simulink model "FOC_Part2"  (R2021b)
settings: Solver=ode45  StartTime=0.0  StopTime=0.2  MaxStep=1e-6  RelTol=1e-3
undefined symbols (not defined in the file): CurKi, CurKp, CurMax, CurTs, F, Id_Target, J, Kt, Ld, Lq, Ls, Mode, Np, Rs, SpdKi, SpdKp, SpdTs, TargetSpd, Tf, Theta_Init, TickAdd, Tn, Udc, VolMax
libraries: spsPermanentMagnetSynchronousMachineLib x1, spsCurrentMeasurementLib x1, spsDCVoltageSourceLib x1, eeGeneralControl x1, spsOnDelayLib x1, simulink x1, spsUniversalBridgeLib x1, spsVoltageMeasurementLib x1, spspowerguiLib x1
settings Model: SimulationMode=accelerator  Creator=LFL  LastModifiedBy=62555
settings SolverCC: AlgebraicLoopSolver=TrustRegion
settings DataIOCC: ReturnWorkspaceOutputs=off
settings DebuggingCC: SFMachineParentedDataDiag=warning  ArithmeticOperatorsInVariantConditions=warning
settings SFSimCC: SimUseLocalCustomCode=off  CustomCodeUndefinedFunction=UseInterfaceOnly
settings RTWCC: RTWUseLocalCustomCode=off

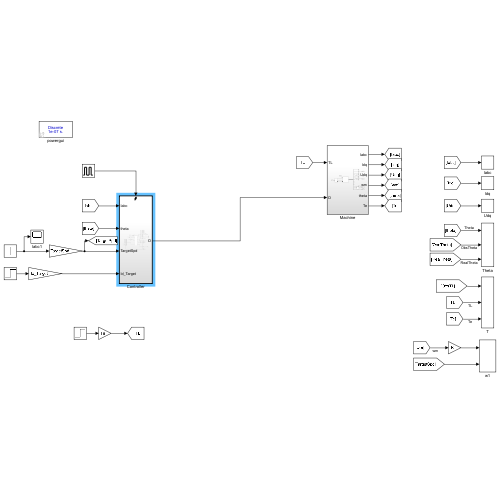
[thumbnail: Simulink's stored preview of the top-level diagram]
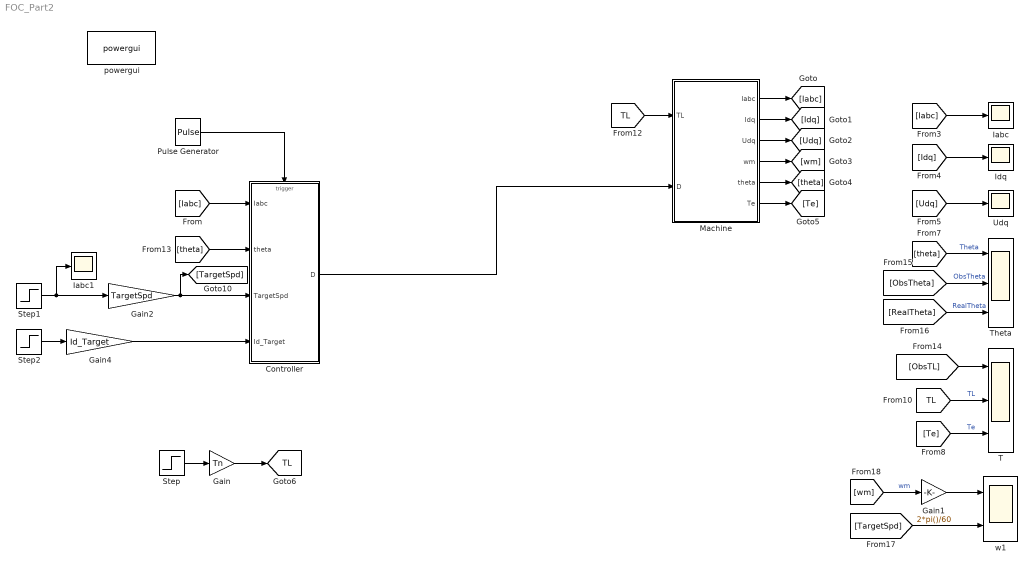
== system FOC_Part2 ==
  Controller : Subsystem  TreatAsAtomicUnit=on
  Gain : Gain  Gain=Tn
  Gain1 : Gain  Gain=2*pi()/60
  Gain2 : Gain  Gain=TargetSpd
  Gain4 : Gain  Gain=Id_Target
  Iabc : Scope
  Iabc1 : Scope
  Idq : Scope
  Machine : Subsystem
  Pulse Generator : DiscretePulseGenerator  PulseType=Time based  Period=CurTs  PulseWidth=50
  Step : Step  Time=0  SampleTime=0
  Step1 : Step  Time=0.1  SampleTime=0
  Step2 : Step  Time=0.1  SampleTime=0
  T : Scope  NumInputPorts=3
  Theta : Scope  NumInputPorts=3
  Udq : Scope
  powergui : spspowerguiLib/powergui  Priority=1  SimulationMode=Discrete  SampleTime=1/500/20000  frequency=60  Iterations=50  frequencyindice=0  Pbase=100e6  ErrMax=1e-4  UnitsV=kV  UnitsW=MW  buscounter=0  FunctionMessages=off  echomessages=off  EnableUseOfTLC=off  CurrentSourceSwitches=off  DisableSnubberDevices=off  DisableRonSwitches=off  DisableVfSwitches=off  DisplayEquations=off  AutomaticDiscreteSolvers=off  SolverType=Tustin/Backward Euler (TBE)  Interpol=off  ExternalGateDelay=off  methode=off  Ts=100  x0status=blocks  SPID=on  SwTol=0  HookPort=off  NonlinearTolerance=1e-4  nMaxIteration=100  ContinueOnMaxIteration=off  RestoreLinks=warning  ResistiveCurrentMeasurement=off  Frange=[0:2:500]  Ylog=off  Xlog=on  ShowGrid=off  save=off  variable=ZData  structure=0  ZoomFFT=off  StartTime=0.0  cycles=1  DisplayStyle=1  fundamental=60  FreqAxis=off  MaxFrequency=1000  frequencyindicesteady=1  RmsSteady=1  display=off
  w1 : Scope  NumInputPorts=2
  tag scope: TL=global
  wires:
  Pulse Generator/1 -> Controller/Trigger
  Machine/1(Iabc) -> [Iabc]
  Machine/2(Idq) -> [Idq]
  Machine/3(Udq) -> [Udq]
  Machine/4(wm) -> [wm]
  Machine/5(theta) -> [theta]
  Machine/6(Te) -> [Te]
  [Iabc] -> Controller/1(Iabc)
  [Iabc] -> Iabc/1
  [Udq] -> Udq/1
  [TL] -> T/2  "TL"
  [Te] -> T/3  "Te"
  [theta] -> Theta/1  "Theta"
  [Idq] -> Idq/1
  [TL] -> Machine/1(TL)
  [theta] -> Controller/2(theta)
  Step/1 -> Gain/1
  Gain/1 -> [TL]
  Controller/1(D) -> Machine/2(D)
  Gain2/1 -> Controller/3(TargetSpd), [TargetSpd]
  [ObsTL] -> T/1
  [ObsTheta] -> Theta/2  "ObsTheta"
  [RealTheta] -> Theta/3  "RealTheta"
  Step1/1 -> Gain2/1, Iabc1/1
  [TargetSpd] -> w1/2
  [wm] -> Gain1/1  "wm"
  Gain1/1 -> w1/1
  Step2/1 -> Gain4/1
  Gain4/1 -> Controller/4(Id_Target)

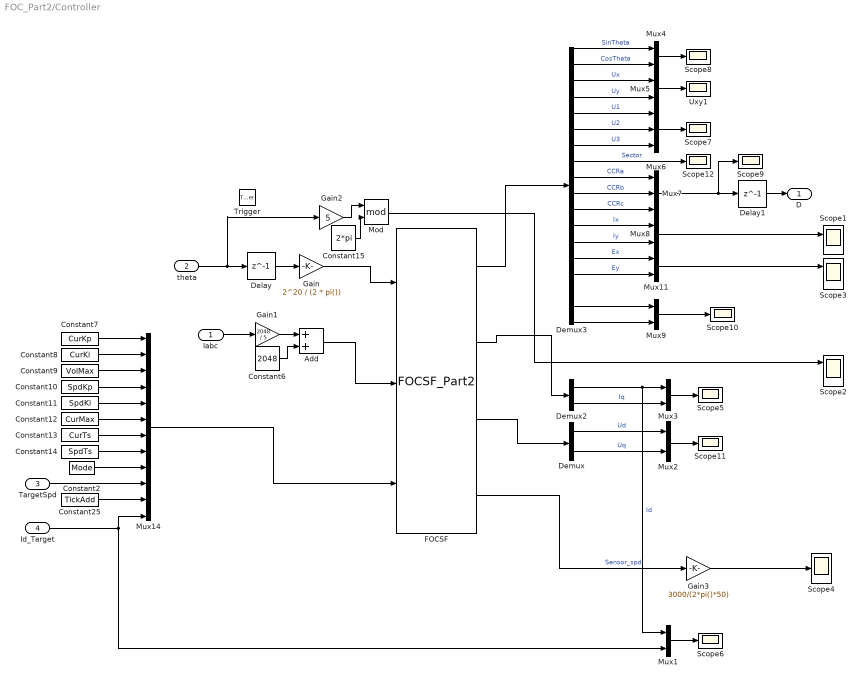
== system FOC_Part2/Controller ==
  Iabc : Inport
  theta : Inport  Port=2
  TargetSpd : Inport  Port=3
  Id_Target : Inport  Port=4
  Trigger : TriggerPort  VariantControl=Variant
  Add : Sum
  Constant10 : Constant  Value=SpdKp
  Constant11 : Constant  Value=SpdKi
  Constant12 : Constant  Value=CurMax
  Constant13 : Constant  Value=CurTs
  Constant14 : Constant  Value=SpdTs
  Constant15 : Constant  Value=2*pi
  Constant2 : Constant  Value=Mode
  Constant25 : Constant  Value=TickAdd
  Constant6 : Constant  Value=2048
  Constant7 : Constant  Value=CurKp
  Constant8 : Constant  Value=CurKi
  Constant9 : Constant  Value=VolMax
  Delay : Delay  DelayLength=1
  Delay1 : Delay  DelayLength=1
  Demux : Demux  Outputs=2
  Demux2 : Demux  Outputs=2
  Demux3 : Demux  Outputs=18
  FOCSF : S-Function  FunctionName=FOCSF_Part2  Parameters=Np Udc Ls Rs Kt J Ld Lq  SFunctionDeploymentMode=off  EnableBusSupport=off  mask{Np=Np, Udc=Udc, Ls=Ls, Rs=Rs, Kt=Kt, J=J, Ld=Ld, Lq=Lq}
      mask Display:
      | port_label('input',  1,  'Theta')
      | port_label('input',  2,  'Iabc')
      | port_label('input',  3,  'CtrlParam')
      | port_label('output', 1,  'FOC')
      | port_label('output', 2,  'Idq')
      | port_label('output', 3,  'Udq')
      | port_label('output', 4,  'Spd')
  Gain : Gain  Gain=2^20 / (2 * pi())
  Gain1 : Gain  Gain=2048 / 5
  Gain2 : Gain  Gain=5
  Gain3 : Gain  Gain=3000/(2*pi()*50)
  Mod : Math  Operator=mod  SaturateOnIntegerOverflow=on
  Mux{1..5,8..9,11} (8 alike) : Mux  Inputs=2
  Mux14 : Mux  Inputs=12
  Mux6 : Mux  Inputs=3
  Mux7 : Mux  Inputs=3
  Scope1 : Scope  NumInputPorts=2
  Scope{4..12} (9 alike) : Scope
  Scope2 : Scope  NumInputPorts=2
  Scope3 : Scope  NumInputPorts=2
  Uxy1 : Scope
  D : Outport  VectorParamsAs1DForOutWhenUnconnected=off
  wires:
  Iabc/1 -> Gain1/1
  Gain/1 -> FOCSF/1
  Gain1/1 -> Add/1
  Constant6/1 -> Add/2
  Add/1 -> FOCSF/2
  theta/1 -> Gain2/1, Delay/1
  Delay/1 -> Gain/1
  FOCSF/2 -> Demux2/1
  FOCSF/3 -> Demux/1
  Demux/1 -> Mux2/1  "Ud"
  Demux/2 -> Mux2/2  "Uq"
  Mux2/1 -> Scope11/1
  Delay1/1 -> D/1
  Demux2/1 -> Mux1/1, Mux3/1  "Id"
  Demux2/2 -> Mux3/2  "Iq"
  Mux3/1 -> Scope5/1
  FOCSF/1 -> Demux3/1
  Demux3/1 -> Mux4/1  "SinTheta"
  Demux3/2 -> Mux4/2  "CosTheta"
  Mux4/1 -> Scope8/1
  Demux3/3 -> Mux5/1  "Ux"
  Demux3/4 -> Mux5/2  "Uy"
  Mux6/1 -> Scope7/1
  Demux3/5 -> Mux6/1  "U1"
  Demux3/6 -> Mux6/2  "U2"
  Demux3/7 -> Mux6/3  "U3"
  Demux3/8 -> Scope12/1  "Sector"
  Demux3/9 -> Mux7/1  "CCRa"
  Demux3/10 -> Mux7/2  "CCRb"
  Demux3/11 -> Mux7/3  "CCRc"
  Mux7/1 -> Scope9/1, Delay1/1
  Demux3/13 -> Mux8/2  "Iy"
  Demux3/12 -> Mux8/1  "Ix"
  Demux3/15 -> Mux11/2  "Ey"
  Demux3/14 -> Mux11/1  "Ex"
  Mux14/1 -> FOCSF/3
  Constant7/1 -> Mux14/1
  Constant8/1 -> Mux14/2
  Constant9/1 -> Mux14/3
  Constant11/1 -> Mux14/5
  Constant10/1 -> Mux14/4
  Constant12/1 -> Mux14/6
  Constant13/1 -> Mux14/7
  Constant14/1 -> Mux14/8
  Constant2/1 -> Mux14/9
  TargetSpd/1 -> Mux14/10
  Constant25/1 -> Mux14/11
  Mux5/1 -> Uxy1/1
  Mux11/1 -> Scope3/1
  Mux8/1 -> Scope1/1
  Gain2/1 -> Mod/1
  Mod/1 -> Scope2/1
  Constant15/1 -> Mod/2
  FOCSF/4 -> Gain3/1  "Sensor_spd"
  Id_Target/1 -> Mux1/2, Mux14/12
  Mux1/1 -> Scope6/1
  Gain3/1 -> Scope4/1
  Demux3/17 -> Mux9/1
  Demux3/18 -> Mux9/2
  Mux9/1 -> Scope10/1

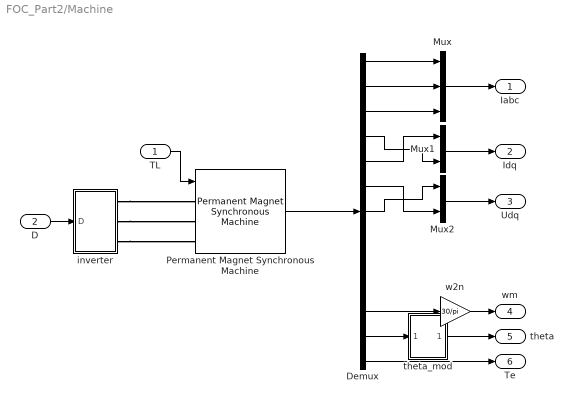
== system FOC_Part2/Machine ==
  TL : Inport
  D : Inport  Port=2
  Demux : Demux  Outputs=13
  Mux : Mux  Inputs=3
  Mux1 : Mux  Inputs=2
  Mux2 : Mux  Inputs=2
  Permanent Magnet Synchronous Machine : spsPermanentMagnetSynchronousMachineLib/Permanent Magnet Synchronous Machine  NbPhases=3  FluxDistribution=Sinusoidal  RotorType=Salient-pole  MechanicalLoad=Torque Tm  PresetModel=No  ShowDetailedParameters=on  MeasurementBus=off  Resistance=Rs  Inductance=8.5e-3  dqInductances=[Ld, Lq]  La=0.000395  MachineConstant=Torque Constant (N.m / A_peak)  Flux=0.014667  VoltageCst=13.3012  TorqueCst=Kt  Flat=120  Mechanical=[J F Np Tf]  PolePairs=4  InitialConditions=[0,Theta_Init, 0,0]  InitialConditions5ph=[0 0 0 0 0 0]  RefAngle=Aligned with phase A axis (original Park)  IterativeDiscreteModel=Trapezoidal non iterative  TsBlock=-1  TsPowergui=0
  inverter : Subsystem
  theta_mod : Subsystem
  w2n : Gain  Gain=30/pi
  Iabc : Outport  VectorParamsAs1DForOutWhenUnconnected=off
  Idq : Outport  Port=2  VectorParamsAs1DForOutWhenUnconnected=off
  Udq : Outport  Port=3  VectorParamsAs1DForOutWhenUnconnected=off
  wm : Outport  Port=4  VectorParamsAs1DForOutWhenUnconnected=off
  theta : Outport  Port=5  VectorParamsAs1DForOutWhenUnconnected=off
  Te : Outport  Port=6  VectorParamsAs1DForOutWhenUnconnected=off
  wires:
  Permanent Magnet Synchronous Machine/1 -> Demux/1
  Demux/1 -> Mux/1
  Demux/2 -> Mux/2
  Demux/3 -> Mux/3
  Mux/1 -> Iabc/1
  Mux1/1 -> Idq/1
  Mux2/1 -> Udq/1
  Demux/11 -> w2n/1
  Demux/12 -> theta_mod/1(In1)
  Demux/13 -> Te/1
  TL/1 -> Permanent Magnet Synchronous Machine/1
  Demux/5 -> Mux1/1
  Demux/4 -> Mux1/2
  Demux/6 -> Mux2/2
  Demux/7 -> Mux2/1
  theta_mod/1(Out1) -> theta/1
  w2n/1 -> wm/1
  D/1 -> inverter/1(D)
  connections:
  inverter/RConn1 -- Permanent Magnet Synchronous Machine/LConn1
  inverter/RConn2 -- Permanent Magnet Synchronous Machine/LConn2
  inverter/RConn3 -- Permanent Magnet Synchronous Machine/LConn3

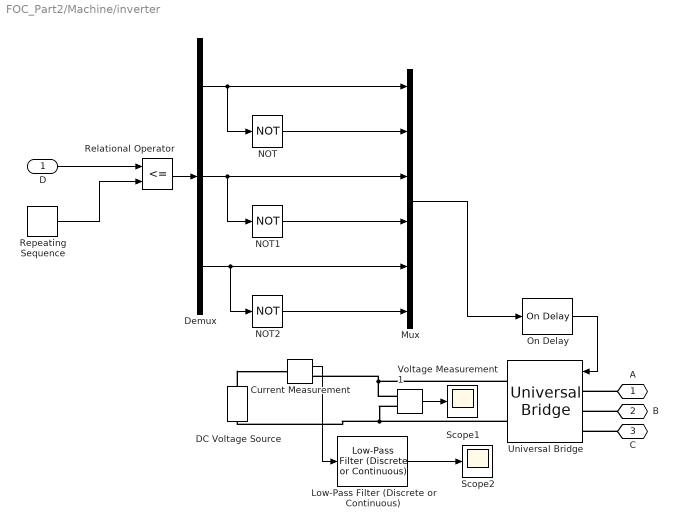
== system FOC_Part2/Machine/inverter ==
  D : Inport
  Current Measurement : spsCurrentMeasurementLib/Current Measurement  PhasorSimulation=off  OutputType=Complex  PSBequivalent=0
  DC Voltage Source : spsDCVoltageSourceLib/DC Voltage Source  Amplitude=Udc  Measurements=None
  Demux : Demux  Outputs=3
  Low-Pass Filter (Discrete or Continuous) : eeGeneralControl/Low-Pass Filter (Discrete or Continuous)  K=1  T=0.01  B=inf  A=-inf  init_option=Inherited from block input  x0=0  Ts=-1
  Mux : Mux  Inputs=6
  NOT : Logic  Operator=NOT  IconShape=distinctive  AllPortsSameDT=off  OutDataTypeStr=boolean
  NOT1 : Logic  Operator=NOT  IconShape=distinctive  AllPortsSameDT=off  OutDataTypeStr=boolean
  NOT2 : Logic  Operator=NOT  IconShape=distinctive  AllPortsSameDT=off  OutDataTypeStr=boolean
  On Delay : spsOnDelayLib/On Delay  DelayType=On delay  delay=Deadtime  ic=0  Ts=0
      settings: SourceProductBaseCode=PS
  Relational Operator : RelationalOperator  Operator=<=  OutDataTypeStr=boolean  RndMeth=Simplest
  Repeating Sequence : simulink/Sources/Repeating Sequence  rep_seq_t=[0 CurTs/2 CurTs]  rep_seq_y=[0 1 0]
  Scope1 : Scope
  Scope2 : Scope
  Universal Bridge : spsUniversalBridgeLib/Universal Bridge  Arms=3  SnubberResistance=1e5  SnubberCapacitance=inf  Device=MOSFET / Diodes  Ron=0.007  Lon=0  ForwardVoltages="[  0  0  ]"  ForwardVoltage=0  GTOparameters=[ 10e-6 , 20e-6 ]  IGBTparameters=[ 1e-6 , 2e-6 ]  Measurements=None  Measurements_2=None  converterType=Rectifier
  Voltage Measurement1 : spsVoltageMeasurementLib/Voltage Measurement  PhasorSimulation=off  OutputType=Complex  PSBequivalent=0
  A : PMIOPort  Side=Right
  B : PMIOPort  Port=2  Side=Right
  C : PMIOPort  Port=3  Side=Right
  wires:
  On Delay/1 -> Universal Bridge/1
  NOT1/1 -> Mux/4
  NOT/1 -> Mux/2
  Demux/1 -> Mux/1, NOT/1
  Demux/3 -> NOT2/1, Mux/5
  Demux/2 -> NOT1/1, Mux/3
  NOT2/1 -> Mux/6
  Relational Operator/1 -> Demux/1
  D/1 -> Relational Operator/1
  Mux/1 -> On Delay/1
  Voltage Measurement1/1 -> Scope1/1
  Current Measurement/1 -> Low-Pass Filter (Discrete or Continuous)/1
  Low-Pass Filter (Discrete or Continuous)/1 -> Scope2/1
  Repeating Sequence/1 -> Relational Operator/2
  connections:
  A/RConn1 -- Universal Bridge/LConn1
  B/RConn1 -- Universal Bridge/LConn2
  C/RConn1 -- Universal Bridge/LConn3
  Universal Bridge/RConn1 -- Current Measurement/RConn1 -- Voltage Measurement1/LConn1
  Voltage Measurement1/LConn2 -- DC Voltage Source/LConn1 -- Universal Bridge/RConn2
  DC Voltage Source/RConn1 -- Current Measurement/LConn1

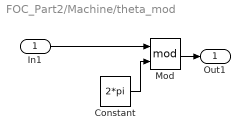
== system FOC_Part2/Machine/theta_mod ==
  In1 : Inport
  Constant : Constant  Value=2*pi
  Mod : Math  Operator=mod  SignedPower=on  SaturateOnIntegerOverflow=on
  Out1 : Outport  VectorParamsAs1DForOutWhenUnconnected=off
  wires:
  Mod/1 -> Out1/1
  Constant/1 -> Mod/2
  In1/1 -> Mod/1
